simulink model "non_linear_simulation"  (R2020a)
settings: Solver=ode4  StartTime=0.0  StopTime=inf  FixedStep=0.01  RelTol=1e-3
libraries: realtime_pacer_lib x1
settings Model: Creator=engen  LastModifiedBy=engen

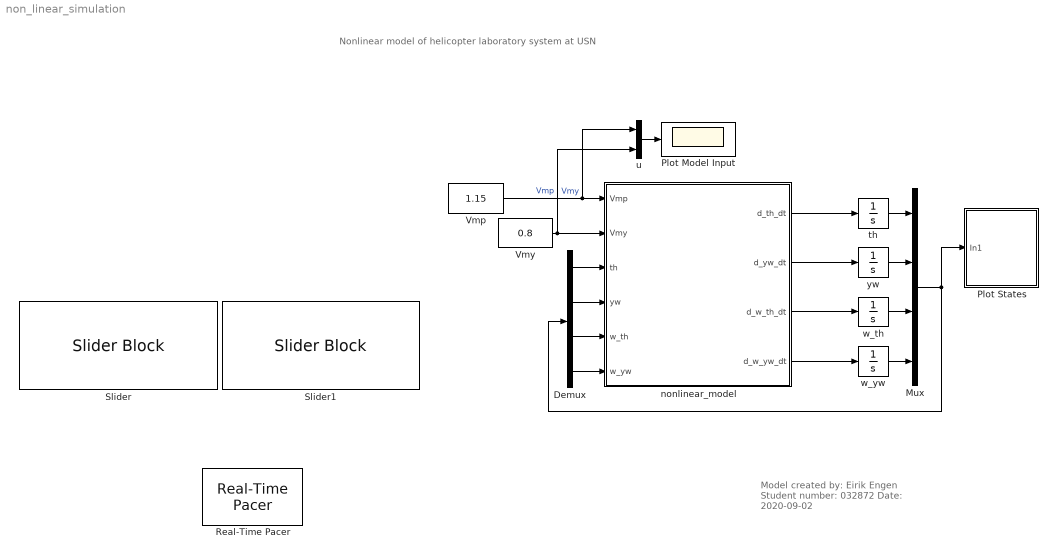
== system non_linear_simulation ==
  note: Model created by: Eirik Engen
      | Student number: 032872
      | Date: 2020-09-02
  note: Nonlinear model of helicopter laboratory system at USN
  Demux : Demux
  Mux : Mux
  Plot Model Input : Scope
  Plot States : Subsystem
  Real-Time Pacer : realtime_pacer_lib/Real-Time Pacer  simTimePerRealTime=1
  Slider : SliderBlock  ScaleMax=1.5
  Slider1 : SliderBlock  ScaleMax=1.5
  Vmp : Constant  Value=1.15  SampleTime=-1
  Vmy : Constant  Value=0.8  SampleTime=-1
  nonlinear_model : MATLAB Function  TreatAsAtomicUnit=on
  th : Integrator  InitialCondition=-45*pi/180  LimitOutput=on  UpperSaturationLimit=45*pi/180  LowerSaturationLimit=-45*pi/180  ContinuousStateAttributes='th'
  u : Mux  Inputs=2
  w_th : Integrator  ContinuousStateAttributes='w_th'
  w_yw : Integrator  ContinuousStateAttributes='w_yw'
  yw : Integrator  LimitOutput=on  UpperSaturationLimit=180*pi/180  LowerSaturationLimit=0  ContinuousStateAttributes='yw'
  wires:
  Vmp/1 -> u/1, nonlinear_model/1(Vmp)  "Vmp"
  Vmy/1 -> u/2, nonlinear_model/2(Vmy)  "Vmy"
  nonlinear_model/1(d_th_dt) -> th/1
  nonlinear_model/2(d_yw_dt) -> yw/1
  nonlinear_model/3(d_w_th_dt) -> w_th/1
  nonlinear_model/4(d_w_yw_dt) -> w_yw/1
  th/1 -> Mux/1
  yw/1 -> Mux/2
  w_th/1 -> Mux/3
  w_yw/1 -> Mux/4
  Mux/1 -> Plot States/1(In1), Demux/1
  Demux/1 -> nonlinear_model/3(th)
  Demux/2 -> nonlinear_model/4(yw)
  Demux/3 -> nonlinear_model/5(w_th)
  Demux/4 -> nonlinear_model/6(w_yw)
  u/1 -> Plot Model Input/1

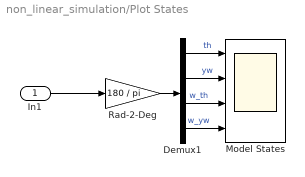
== system non_linear_simulation/Plot States ==
  In1 : Inport
  Demux1 : Demux
  Model States : Scope  NumInputPorts=4
  Rad-2-Deg : Gain  Gain=180 / pi
  wires:
  In1/1 -> Rad-2-Deg/1
  Demux1/2 -> Model States/2  "yw"
  Demux1/3 -> Model States/3  "w_th"
  Demux1/1 -> Model States/1  "th"
  Demux1/4 -> Model States/4  "w_yw"
  Rad-2-Deg/1 -> Demux1/1

== matlab function non_linear_simulation/nonlinear_model ==
  data: Vmp input; d_th_dt output; Vmy input; th input; yw input; w_th input; w_yw input; d_yw_dt output; d_w_th_dt output; d_w_yw_dt output
% Simulink nonlinear model of USN helicopter
% Author: Eirik Engen
% Date: 2020-09-02

function [d_th_dt, d_yw_dt, d_w_th_dt, d_w_yw_dt] = non_linear_model(Vmp, Vmy, th, yw, w_th, w_yw)          %#ok<INUSL>
% function inputs
% Vmp : Model input - Voltage input to Pitch motor/rotor [V]
% Vmy : Model input - Voltage input to Yaw motor/rotor [V]
% th  : Model state - Pitch angle, theta [radians]
% yw  : Model state - Yaw angle, psi [radians]
% w_th: Model state - Pitch angular velocity, omega_theta [radians / s]
% w_yw: Model state - Yaw angular velocity, omega_psi [radians / s]

% System parameters
l_cm   = 0.015;   % [m] - Distance between the pivot point and the center of mass of the helicopter.
m_heli = 0.479;   % [kg] - Total moving mass of the helicopter
J_eq_p = 0.0172;  % [kg-m^2] - Moment of inertia about pitch axis
J_eq_y = 0.0210;  % [kg-m^2] - Moment of inertia about yaw axis
g      = 9.81;    % [m/s^2] - Acceleration due to gravity on planet earth

Kpp    = 0.0556;  % [Nm/V] - Torque constant on pitch axis from pitch motor
Kyy    = 0.21084; % [Nm/V] - Torque constant on yaw axis from yaw motor
Kpy    = 0.005;   % [Nm/V] - Torque constant on pitch axis from yaw motor
Kyp    = 0.15;    % [Nm/V] - Torque constant on yaw axis from pitch motor
Bp     = 0.01;    % [N/V]  - Damping friction factor about pitch axis
By     = 0.08;    % [N/V]  - Damping friction factor about yaw axis

% Differential equations
d_th_dt = w_th;
d_yw_dt = w_yw;
d_w_th_dt = (Kpp*Vmp - ...
    Kpy*Vmy - ...
    Bp*w_th - ...
    m_heli*l_cm^2*w_yw^2*sin(th)*cos(th) - ...
    m_heli*g*l_cm*cos(th)) / ...
    (J_eq_p+m_heli*l_cm^2);
d_w_yw_dt = (Kyp*Vmp - ...
    Kyy*Vmy - ...
    By*w_yw + ...
    2*m_heli*l_cm^2*w_th*w_yw*sin(th)*cos(th)) / ...
    (J_eq_y+m_heli*l_cm^2*cos(th)^2);
